simulink model "sm_pd"  (R2025b)
settings: Solver=VariableStepAuto  StartTime=0.0  StopTime=10.0  RelTol=1e-3
libraries: cstblocks x1
settings Model: Creator=AIZAZ BADRU  LastModifiedBy=AIZAZ BADRU

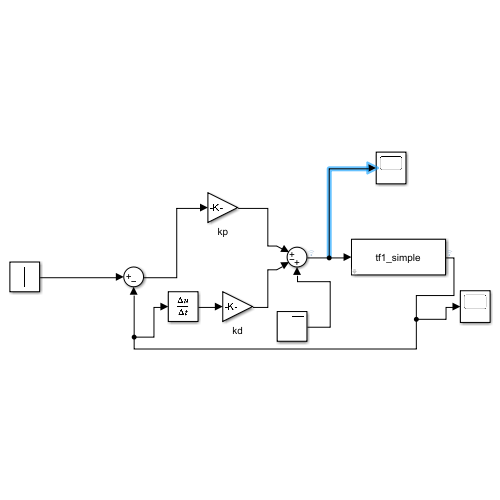
[thumbnail: Simulink's stored preview of the top-level diagram]
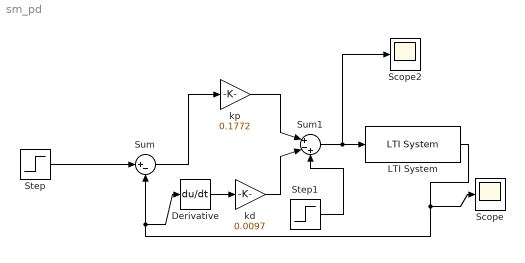
== system sm_pd ==
  Derivative : Derivative
  LTI System : cstblocks/LTI System  sys=tf1_simple  IC=[]  PadeOrder=0
  Scope : Scope
      settings: ActiveDisplayYMinimum=-16.027021823103308  ActiveDisplayYMaximum=144.24319640792982
  Scope2 : Scope
      settings: ActiveDisplayYMinimum=-5.3791905834535454  ActiveDisplayYMaximum=46.976520753979273  DataLoggingVariableName=ScopeData2
  Step : Step  Time=0  After=100  SampleTime=0
  Step1 : Step  Time=4  After=5  SampleTime=0
  Sum : Sum  Inputs=|+-
  Sum1 : Sum  Inputs=|+-+
  kd : Gain  Gain=0.0097
  kp : Gain  Gain=0.1772
  wires:
  LTI System/1 -> Derivative/1, Sum/2, Scope/1
  Sum1/1 -> Scope2/1, LTI System/1
  Sum/1 -> kp/1
  kp/1 -> Sum1/1
  Derivative/1 -> kd/1
  Step/1 -> Sum/1
  kd/1 -> Sum1/2
  Step1/1 -> Sum1/3
